simulink model "Celsisu_to_fahreinheit_subsystem"  (R2020b)
settings: Solver=VariableStepAuto  StartTime=0.0  StopTime=10.0  RelTol=1e-3
libraries: simulink_extras x1, simulink x1
settings Model: Creator=C-TEA  LastModifiedBy=C-TEA

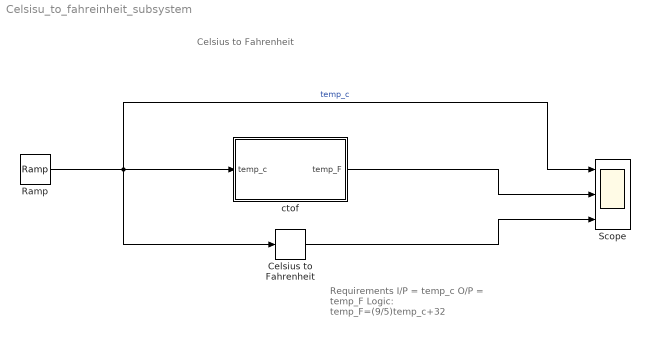
== system Celsisu_to_fahreinheit_subsystem ==
  note: Requirements
      | I/P = temp_c
      | O/P = temp_F
      | Logic: temp_F=(9/5)temp_c+32
  note: Celsius to Fahrenheit
  Celsius to Fahrenheit : simulink_extras/Transformations/Celsius to Fahrenheit
      settings: SourceProductBaseCode=SL
  Ramp : simulink/Sources/Ramp  slope=1  start=0  InitialOutput=0
  Scope : Scope  NumInputPorts=3
  ctof : Subsystem
  wires:
  Ramp/1 -> Scope/1, Celsius to Fahrenheit/1, ctof/1(temp_c)  "temp_c"
  Celsius to Fahrenheit/1 -> Scope/3
  ctof/1(temp_F) -> Scope/2

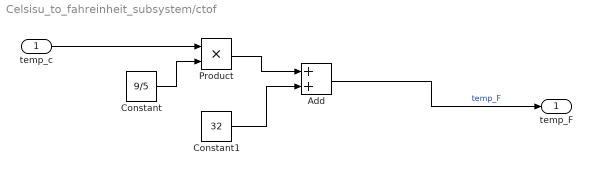
== system Celsisu_to_fahreinheit_subsystem/ctof ==
  temp_c : Inport
  Add : Sum
  Constant : Constant  Value=9/5
  Constant1 : Constant  Value=32
  Product : Product
  temp_F : Outport
  wires:
  Product/1 -> Add/1
  Constant/1 -> Product/2
  Constant1/1 -> Add/2
  Add/1 -> temp_F/1  "temp_F"
  temp_c/1 -> Product/1
